simulink model "mrefrobotarm_modified_previous_y_previous_u_previous_ref_pert_2"  (R2018b)
settings: Solver=FixedStepAuto  StartTime=0.0  StopTime=60  RelTol=1e-3  AbsTol=1e-6
undefined symbols (not defined in the file or in its folder): cc, options
libraries: neural x858, simulink x1
(part 16 of 32)

== system mrefrobotarm_modified_previous_y_previous_u_previous_ref_pert_2/m=0 sd=0.1/Layer 3/Delays 1 ==
  "p{3}" : Inport  PortDimensions=30
      mask Display: e = 0.06;c1 = [120 230 180]/255;c2 = ([120 230 180]+0)/(256+128);c3 = ([120 230 180]+128)/(256+128);patch([0 1 1 0],[0 0 1 1],c1);patch([0 1 1 1-e 1-e 0+e],[0 0 1 1-e 0+e 0+e],c2);patch([0 0 1 1-e 0+e 0+e],[0 1 1 1-e 1-e 0+e],c3);plot([0 1 1 0 0],[0 0 1 1 0]);
  mux : Mux  Inputs=1
      mask Display: e = 0.06;c1 = [120 150 230]/255;c2 = ([120 150 230]+0)/383;c3 = ([120 150 230]+128)/383;patch([0 1 1 0],[0 0 1 1],c1);patch([0 1 1 1-e 1-e 0+e],[0 0 1 1-e 0+e 0+e],c2);patch([0 0 1 1-e 0+e 0+e],[0 1 1 1-e 1-e 0+e],c3);plot([0 1 1 0 0],[0 0 1 1 0]);disp('Mux')
  "pd{3,2}" : Outport
      mask Display: e = 0.06;c1 = [120 230 180]/255;c2 = ([120 230 180]+0)/(256+128);c3 = ([120 230 180]+128)/(256+128);patch([0 1 1 0],[0 0 1 1],c1);patch([0 1 1 1-e 1-e 0+e],[0 0 1 1-e 0+e 0+e],c2);patch([0 0 1 1-e 0+e 0+e],[0 1 1 1-e 1-e 0+e],c3);plot([0 1 1 0 0],[0 0 1 1 0]);
  wires:
  "p{3}"/1 -> mux/1
  mux/1 -> "pd{3,2}"/1

== system mrefrobotarm_modified_previous_y_previous_u_previous_ref_pert_2/m=0 sd=0.1/Layer 3/LW{3,2} ==
  "ad{3,2}" : Inport  PortDimensions=30
      mask Display: e = 0.06;c1 = [120 230 180]/255;c2 = ([120 230 180]+0)/(256+128);c3 = ([120 230 180]+128)/(256+128);patch([0 1 1 0],[0 0 1 1],c1);patch([0 1 1 1-e 1-e 0+e],[0 0 1 1-e 0+e 0+e],c2);patch([0 0 1 1-e 0+e 0+e],[0 1 1 1-e 1-e 0+e],c3);plot([0 1 1 0 0],[0 0 1 1 0]);
  "IW{3,2}(1,:)'" : Constant  Value=[0.55901254797417976316609156128834001719951629638671875;0.1893376853911200308200335484798415564000606536865234375;-0.0561053598569281330998848034141701646149158477783203125;0.006936116057090567499354705205405480228364467620849609375;0.10585635712547609987854713153865304775536060333251953125;-0.056411161009771886021280096201735432259738445281982421875;-0.362521364744238516752972145695821382105350494384765625;0.061274149008166800545183150461525656282901763916015625;-0.10299753787049596709390897331104497425258159637451171875;-1.0111912490182943802352610873640514910221099853515625;0.0080365135532425302500314501230604946613311767578125;0.038057999796948550896846796831596293486654758453369140625;0.0182019329420017549059362949037677026353776454925537109375;0.000718748845277970729687744277924821290071122348308563232421875;-0.0892154937366842204493622148220310918986797332763671875;0.04086688119049319833919753364170901477336883544921875;0.07794534518223993069252486520781530998647212982177734375;0.00118864659777381700793419394557304258341901004314422607421875;0.2021661306486308429253284657534095458686351776123046875;0.03908324016475679674176291200637933798134326934814453125;-0.088708253793172653356435830573900602757930755615234375;0.0043019444601169846975619037721116910688579082489013671875;-0.417578792656369823799167306788149289786815643310546875;0.0038865187767530167718688094424805967719294130802154541015625;-0.00952243697565639639346368738870296510867774486541748046875;0.416065824298875563957977874451898969709873199462890625;-0.1244373729702374087313643258312367834150791168212890625;0.021685469644277984013758242554104072041809558868408203125;-0.33337725597607625882545789863797836005687713623046875;-0.07267474571307540320841411585206515155732631683349609375]
      mask Display: e = 0.06;c1 = [120 150 230]/255;c2 = ([120 150 230]+0)/383;c3 = ([120 150 230]+128)/383;patch([0 1 1 0],[0 0 1 1],c1);patch([0 1 1 1-e 1-e 0+e],[0 0 1 1-e 0+e 0+e],c2);patch([0 0 1 1-e 0+e 0+e],[0 1 1 1-e 1-e 0+e],c3);plot([0 1 1 0 0],[0 0 1 1 0]);disp('weights');
  Mux : Mux  Inputs=1
      mask Display: e = 0.06;c1 = [120 150 230]/255;c2 = ([120 150 230]+0)/383;c3 = ([120 150 230]+128)/383;patch([0 1 1 0],[0 0 1 1],c1);patch([0 1 1 1-e 1-e 0+e],[0 0 1 1-e 0+e 0+e],c2);patch([0 0 1 1-e 0+e 0+e],[0 1 1 1-e 1-e 0+e],c3);plot([0 1 1 0 0],[0 0 1 1 0]);disp('Mux');
  dotprod1 : neural/Weight Functions/dotprod
  "lz{3,2}" : Outport
      mask Display: e = 0.06;c1 = [120 230 180]/255;c2 = ([120 230 180]+0)/(256+128);c3 = ([120 230 180]+128)/(256+128);patch([0 1 1 0],[0 0 1 1],c1);patch([0 1 1 1-e 1-e 0+e],[0 0 1 1-e 0+e 0+e],c2);patch([0 0 1 1-e 0+e 0+e],[0 1 1 1-e 1-e 0+e],c3);plot([0 1 1 0 0],[0 0 1 1 0]);
  wires:
  "IW{3,2}(1,:)'"/1 -> dotprod1/1
  "ad{3,2}"/1 -> dotprod1/2
  dotprod1/1 -> Mux/1
  Mux/1 -> "lz{3,2}"/1

== system mrefrobotarm_modified_previous_y_previous_u_previous_ref_pert_2/m=0 sd=0.2/Layer 1/Delays 1 ==
  "p{1}" : Inport  PortDimensions=10
      mask Display: e = 0.06;c1 = [120 230 180]/255;c2 = ([120 230 180]+0)/(256+128);c3 = ([120 230 180]+128)/(256+128);patch([0 1 1 0],[0 0 1 1],c1);patch([0 1 1 1-e 1-e 0+e],[0 0 1 1-e 0+e 0+e],c2);patch([0 0 1 1-e 0+e 0+e],[0 1 1 1-e 1-e 0+e],c3);plot([0 1 1 0 0],[0 0 1 1 0]);
  mux : Mux  Inputs=1
      mask Display: e = 0.06;c1 = [120 150 230]/255;c2 = ([120 150 230]+0)/383;c3 = ([120 150 230]+128)/383;patch([0 1 1 0],[0 0 1 1],c1);patch([0 1 1 1-e 1-e 0+e],[0 0 1 1-e 0+e 0+e],c2);patch([0 0 1 1-e 0+e 0+e],[0 1 1 1-e 1-e 0+e],c3);plot([0 1 1 0 0],[0 0 1 1 0]);disp('Mux')
  "pd{1,1}" : Outport
      mask Display: e = 0.06;c1 = [120 230 180]/255;c2 = ([120 230 180]+0)/(256+128);c3 = ([120 230 180]+128)/(256+128);patch([0 1 1 0],[0 0 1 1],c1);patch([0 1 1 1-e 1-e 0+e],[0 0 1 1-e 0+e 0+e],c2);patch([0 0 1 1-e 0+e 0+e],[0 1 1 1-e 1-e 0+e],c3);plot([0 1 1 0 0],[0 0 1 1 0]);
  wires:
  "p{1}"/1 -> mux/1
  mux/1 -> "pd{1,1}"/1

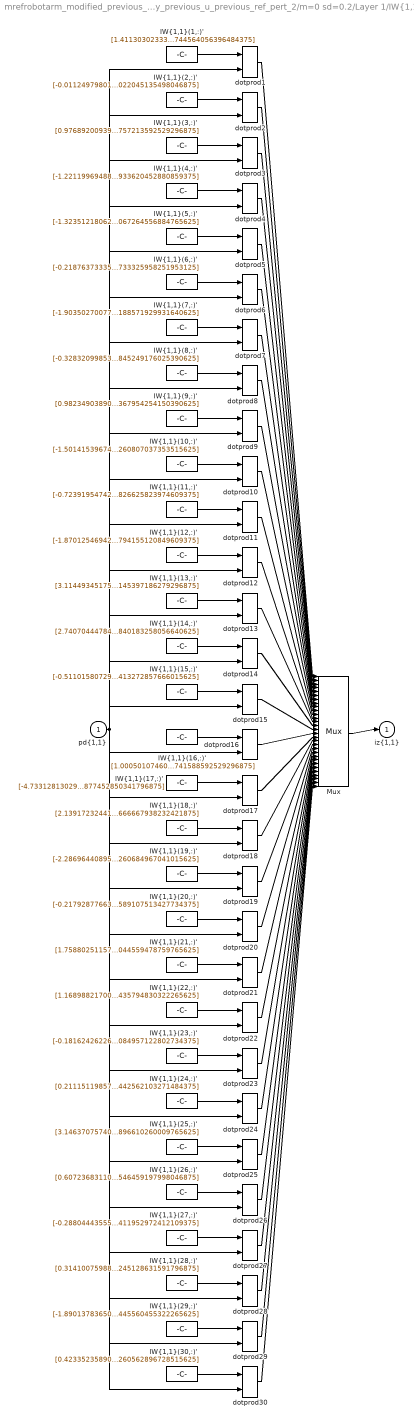
== system mrefrobotarm_modified_previous_y_previous_u_previous_ref_pert_2/m=0 sd=0.2/Layer 1/IW{1,1} ==
  "pd{1,1}" : Inport  PortDimensions=10
      mask Display: e = 0.06;c1 = [120 230 180]/255;c2 = ([120 230 180]+0)/(256+128);c3 = ([120 230 180]+128)/(256+128);patch([0 1 1 0],[0 0 1 1],c1);patch([0 1 1 1-e 1-e 0+e],[0 0 1 1-e 0+e 0+e],c2);patch([0 0 1 1-e 0+e 0+e],[0 1 1 1-e 1-e 0+e],c3);plot([0 1 1 0 0],[0 0 1 1 0]);
  "IW{1,1}(1,:)'" : Constant  Value=[1.4113030233343781816301998333074152469635009765625;-0.348438589909515428200137421299587003886699676513671875;-1.525310697435914963904224350699223577976226806640625;0.2209845967001718702871215782579383812844753265380859375;-0.90644875404291724851901790316333062946796417236328125;3.15955488668658812656531154061667621135711669921875;-1.645213986417652929361565838917158544063568115234375;0.31425769225662125716524997187661938369274139404296875;5.8448616430047390934987561195157468318939208984375;2.639470335514532361997908083139918744564056396484375]
      mask Display: e = 0.06;c1 = [120 150 230]/255;c2 = ([120 150 230]+0)/383;c3 = ([120 150 230]+128)/383;patch([0 1 1 0],[0 0 1 1],c1);patch([0 1 1 1-e 1-e 0+e],[0 0 1 1-e 0+e 0+e],c2);patch([0 0 1 1-e 0+e 0+e],[0 1 1 1-e 1-e 0+e],c3);plot([0 1 1 0 0],[0 0 1 1 0]);disp('Weights');
  "IW{1,1}(10,:)'" : Constant  Value=[-1.5014153967441250525638452018029056489467620849609375;0.9736603972080974944702802531537599861621856689453125;-1.37313114935890911993965346482582390308380126953125;0.453944962788460470992646378363133408129215240478515625;-0.517586043869458389821147648035548627376556396484375;0.86773315026872366306776029887259937822818756103515625;-0.11243588136571429358934182118900935165584087371826171875;0.539938227324440855880993694881908595561981201171875;0.6911668193214997035767055422184057533740997314453125;-0.034160834851410117052328274667161167599260807037353515625]
      mask Display: e = 0.06;c1 = [120 150 230]/255;c2 = ([120 150 230]+0)/383;c3 = ([120 150 230]+128)/383;patch([0 1 1 0],[0 0 1 1],c1);patch([0 1 1 1-e 1-e 0+e],[0 0 1 1-e 0+e 0+e],c2);patch([0 0 1 1-e 0+e 0+e],[0 1 1 1-e 1-e 0+e],c3);plot([0 1 1 0 0],[0 0 1 1 0]);disp('Weights');
  "IW{1,1}(11,:)'" : Constant  Value=[-0.72391954742164899005985034818877466022968292236328125;0.60057208214730983808493647302384488284587860107421875;-1.4507267854128438333560779938125051558017730712890625;0.456866710462218217347896143110119737684726715087890625;0.1570974108836583338355552541543147526681423187255859375;0.733544275114982990970702303457073867321014404296875;-0.598466107260065438566698503564111888408660888671875;-0.480699831251547526900225193458027206361293792724609375;2.35513038112840877857934174244292080402374267578125;1.419047822295259830838176640099845826625823974609375]
      mask Display: e = 0.06;c1 = [120 150 230]/255;c2 = ([120 150 230]+0)/383;c3 = ([120 150 230]+128)/383;patch([0 1 1 0],[0 0 1 1],c1);patch([0 1 1 1-e 1-e 0+e],[0 0 1 1-e 0+e 0+e],c2);patch([0 0 1 1-e 0+e 0+e],[0 1 1 1-e 1-e 0+e],c3);plot([0 1 1 0 0],[0 0 1 1 0]);disp('Weights');
  "IW{1,1}(12,:)'" : Constant  Value=[-1.87012546942036284036703364108689129352569580078125;1.3084444749908488159206854106741957366466522216796875;-1.1877577962136418587846264927065931260585784912109375;1.2551744503796522511862576720886863768100738525390625;0.11790915105610698387916812635012320242822170257568359375;-0.4054577111017920731939057077397592365741729736328125;0.86175101157558942066572171825100667774677276611328125;0.84046199333763393912732908574980683624744415283203125;-1.552570172382738977745475494884885847568511962890625;-0.8322997096343731637801965916878543794155120849609375]
      mask Display: e = 0.06;c1 = [120 150 230]/255;c2 = ([120 150 230]+0)/383;c3 = ([120 150 230]+128)/383;patch([0 1 1 0],[0 0 1 1],c1);patch([0 1 1 1-e 1-e 0+e],[0 0 1 1-e 0+e 0+e],c2);patch([0 0 1 1-e 0+e 0+e],[0 1 1 1-e 1-e 0+e],c3);plot([0 1 1 0 0],[0 0 1 1 0]);disp('Weights');
  "IW{1,1}(13,:)'" : Constant  Value=[3.11449345175705349930694865179248154163360595703125;-3.732348373191891166555933523341082036495208740234375;-0.6723234936499988823044304808718152344226837158203125;1.0218838198423327856545483882655389606952667236328125;0.1369109814135320013495089597199694253504276275634765625;-0.76304172975338036000181318740942515432834625244140625;0.7623366887407232450613037144648842513561248779296875;1.02980844388660042199035160592757165431976318359375;-3.248414372584246923025830255937762558460235595703125;-2.232600966299432609929453974473290145397186279296875]
      mask Display: e = 0.06;c1 = [120 150 230]/255;c2 = ([120 150 230]+0)/383;c3 = ([120 150 230]+128)/383;patch([0 1 1 0],[0 0 1 1],c1);patch([0 1 1 1-e 1-e 0+e],[0 0 1 1-e 0+e 0+e],c2);patch([0 0 1 1-e 0+e 0+e],[0 1 1 1-e 1-e 0+e],c3);plot([0 1 1 0 0],[0 0 1 1 0]);disp('Weights');
  "IW{1,1}(14,:)'" : Constant  Value=[2.74070444784985323138926105457358062267303466796875;-2.820073129625178420809561430360190570354461669921875;-1.1487312568141889723705162396072410047054290771484375;0.088073813383340804339383112164796330034732818603515625;0.49531928111860723529247252372442744672298431396484375;3.474324634455964844192976670456118881702423095703125;-2.657024722837350250159715869813226163387298583984375;-0.0478319365917047878422607709580915980041027069091796875;4.809776553517846053864559507928788661956787109375;5.53419618962490122981989770778454840183258056640625]
      mask Display: e = 0.06;c1 = [120 150 230]/255;c2 = ([120 150 230]+0)/383;c3 = ([120 150 230]+128)/383;patch([0 1 1 0],[0 0 1 1],c1);patch([0 1 1 1-e 1-e 0+e],[0 0 1 1-e 0+e 0+e],c2);patch([0 0 1 1-e 0+e 0+e],[0 1 1 1-e 1-e 0+e],c3);plot([0 1 1 0 0],[0 0 1 1 0]);disp('Weights');
  "IW{1,1}(15,:)'" : Constant  Value=[-0.511015807291060664141468805610202252864837646484375;-0.347029031123842646167076964047737419605255126953125;-0.1718418816922243907985290434226044453680515289306640625;0.55723542002860548816300934049650095403194427490234375;1.001218620463129038711258544935844838619232177734375;0.5480449416585952970848438781104050576686859130859375;-1.2905089839227572579005709485500119626522064208984375;-0.311064951952224777453892556877690367400646209716796875;1.605461938449392444994145989767275750637054443359375;0.57757524693824591199842188871116377413272857666015625]
      mask Display: e = 0.06;c1 = [120 150 230]/255;c2 = ([120 150 230]+0)/383;c3 = ([120 150 230]+128)/383;patch([0 1 1 0],[0 0 1 1],c1);patch([0 1 1 1-e 1-e 0+e],[0 0 1 1-e 0+e 0+e],c2);patch([0 0 1 1-e 0+e 0+e],[0 1 1 1-e 1-e 0+e],c3);plot([0 1 1 0 0],[0 0 1 1 0]);disp('Weights');
  "IW{1,1}(16,:)'" : Constant  Value=[1.000501074609136065163284001755528151988983154296875;-0.71026830395794637862394438343471847474575042724609375;0.56643772389824775803646161875803954899311065673828125;-1.718593345145298822984614162123762071132659912109375;-0.04658830456743641434957936553473700769245624542236328125;1.896992873999785000904694243217818439006805419921875;-1.314207523734456817265936479088850319385528564453125;-0.58100817248522618196915345833986066281795501708984375;6.11342037772077606661014215205796062946319580078125;4.26490922194190869021213075029663741588592529296875]
      mask Display: e = 0.06;c1 = [120 150 230]/255;c2 = ([120 150 230]+0)/383;c3 = ([120 150 230]+128)/383;patch([0 1 1 0],[0 0 1 1],c1);patch([0 1 1 1-e 1-e 0+e],[0 0 1 1-e 0+e 0+e],c2);patch([0 0 1 1-e 0+e 0+e],[0 1 1 1-e 1-e 0+e],c3);plot([0 1 1 0 0],[0 0 1 1 0]);disp('Weights');
  "IW{1,1}(17,:)'" : Constant  Value=[-4.73312813029816314980280367308296263217926025390625;6.01312541072434303401905708597041666507720947265625;0.1446975706664820615632294220631592907011508941650390625;-1.3734916538271806363269433859386481344699859619140625;-0.374570868930040601352260409839800558984279632568359375;-6.0102833405435394098503820714540779590606689453125;5.72011522082058210258992403396405279636383056640625;0.129537853146572012885684443972422741353511810302734375;-17.05733403236849454742696252651512622833251953125;-12.2512694254419596262550840037874877452850341796875]
      mask Display: e = 0.06;c1 = [120 150 230]/255;c2 = ([120 150 230]+0)/383;c3 = ([120 150 230]+128)/383;patch([0 1 1 0],[0 0 1 1],c1);patch([0 1 1 1-e 1-e 0+e],[0 0 1 1-e 0+e 0+e],c2);patch([0 0 1 1-e 0+e 0+e],[0 1 1 1-e 1-e 0+e],c3);plot([0 1 1 0 0],[0 0 1 1 0]);disp('Weights');
  "IW{1,1}(18,:)'" : Constant  Value=[2.139172324417781823058248846791684627532958984375;-1.516704379288808635095620047650299966335296630859375;-0.97354754756783012936693921801634132862091064453125;2.15205674059551288479497088701464235782623291015625;-1.16111579032775669162447229609824717044830322265625;-1.30932797370402465020333693246357142925262451171875;0.4970822382713446785373889724723994731903076171875;0.003946372609830076268189191779356406186707317829132080078125;-1.6373923459250760981120720316539518535137176513671875;-0.876724016447773646376617762143723666667938232421875]
      mask Display: e = 0.06;c1 = [120 150 230]/255;c2 = ([120 150 230]+0)/383;c3 = ([120 150 230]+128)/383;patch([0 1 1 0],[0 0 1 1],c1);patch([0 1 1 1-e 1-e 0+e],[0 0 1 1-e 0+e 0+e],c2);patch([0 0 1 1-e 0+e 0+e],[0 1 1 1-e 1-e 0+e],c3);plot([0 1 1 0 0],[0 0 1 1 0]);disp('Weights');
  "IW{1,1}(19,:)'" : Constant  Value=[-2.2869644089557112920374493114650249481201171875;2.06966810652304555873115532449446618556976318359375;1.90142951742451060681560193188488483428955078125;-0.574308612498034332105589783168397843837738037109375;-0.247708051032199449981163752454449422657489776611328125;0.5564187144200676282679296491551212966442108154296875;-1.56539549833531221878502037725411355495452880859375;0.375078818331078533976352673562359996140003204345703125;2.397843513239210633258835514425300061702728271484375;1.3119695913197606529365657479502260684967041015625]
      mask Display: e = 0.06;c1 = [120 150 230]/255;c2 = ([120 150 230]+0)/383;c3 = ([120 150 230]+128)/383;patch([0 1 1 0],[0 0 1 1],c1);patch([0 1 1 1-e 1-e 0+e],[0 0 1 1-e 0+e 0+e],c2);patch([0 0 1 1-e 0+e 0+e],[0 1 1 1-e 1-e 0+e],c3);plot([0 1 1 0 0],[0 0 1 1 0]);disp('Weights');
  "IW{1,1}(2,:)'" : Constant  Value=[-0.0112497980128958285916951354010961949825286865234375;0.06194588216941789016178887550267972983419895172119140625;0.5652958623659614101342185676912777125835418701171875;-1.180785608869924896424663529614917933940887451171875;0.088823412488288344679432384509709663689136505126953125;2.13880595730649947228130258736200630664825439453125;-2.27945305012616472595254890620708465576171875;0.281685433695026576916831118069239892065525054931640625;4.35874409348693614418834840762428939342498779296875;3.18642541802911960502342481049709022045135498046875]
      mask Display: e = 0.06;c1 = [120 150 230]/255;c2 = ([120 150 230]+0)/383;c3 = ([120 150 230]+128)/383;patch([0 1 1 0],[0 0 1 1],c1);patch([0 1 1 1-e 1-e 0+e],[0 0 1 1-e 0+e 0+e],c2);patch([0 0 1 1-e 0+e 0+e],[0 1 1 1-e 1-e 0+e],c3);plot([0 1 1 0 0],[0 0 1 1 0]);disp('Weights');
  "IW{1,1}(20,:)'" : Constant  Value=[-0.217928776638212584604303856394835747778415679931640625;0.40520405266274883704369358383701182901859283447265625;-0.04396564242946267297984519473175168968737125396728515625;-0.043313894632832923570209260333285783417522907257080078125;-0.045148919419630346994143366146090556867420673370361328125;-0.2359067249724053905168830169714055955410003662109375;0.09766924760321415988073567859828472137451171875;0.0686057321137425735191328612927463836967945098876953125;-0.35078030086031863898909932686365209519863128662109375;-0.3633796929059707192521955221309326589107513427734375]
      mask Display: e = 0.06;c1 = [120 150 230]/255;c2 = ([120 150 230]+0)/383;c3 = ([120 150 230]+128)/383;patch([0 1 1 0],[0 0 1 1],c1);patch([0 1 1 1-e 1-e 0+e],[0 0 1 1-e 0+e 0+e],c2);patch([0 0 1 1-e 0+e 0+e],[0 1 1 1-e 1-e 0+e],c3);plot([0 1 1 0 0],[0 0 1 1 0]);disp('Weights');
  "IW{1,1}(21,:)'" : Constant  Value=[1.7588025115735634873459503069170750677585601806640625;-2.282420941548847448387959957472048699855804443359375;-1.0294915097698116301927484528278000652790069580078125;1.8482290099310336728422043961472809314727783203125;-0.2097696977909766780090450311035965569317340850830078125;-1.9311459400257862117911145105608738958835601806640625;3.31019261230273986740257896599359810352325439453125;-0.417497660482693933037268152475007809698581695556640625;-7.56322499549997484535879266331903636455535888671875;-4.4413848237048316747177523211576044559478759765625]
      mask Display: e = 0.06;c1 = [120 150 230]/255;c2 = ([120 150 230]+0)/383;c3 = ([120 150 230]+128)/383;patch([0 1 1 0],[0 0 1 1],c1);patch([0 1 1 1-e 1-e 0+e],[0 0 1 1-e 0+e 0+e],c2);patch([0 0 1 1-e 0+e 0+e],[0 1 1 1-e 1-e 0+e],c3);plot([0 1 1 0 0],[0 0 1 1 0]);disp('Weights');
  "IW{1,1}(22,:)'" : Constant  Value=[1.168988217006086127724984180531464517116546630859375;-1.732957486285161774475227502989582717418670654296875;1.05320711434076752510691221687011420726776123046875;-0.58838238416820487497460590020637027919292449951171875;1.3083920626301372980293535874807275831699371337890625;1.3241783743371711157266190639347769320011138916015625;-0.6789672752525373056187163456343114376068115234375;-0.05675259587550791906540581521767308004200458526611328125;1.7931659248481632840110933102550916373729705810546875;1.2789209238231313836564595476374961435794830322265625]
      mask Display: e = 0.06;c1 = [120 150 230]/255;c2 = ([120 150 230]+0)/383;c3 = ([120 150 230]+128)/383;patch([0 1 1 0],[0 0 1 1],c1);patch([0 1 1 1-e 1-e 0+e],[0 0 1 1-e 0+e 0+e],c2);patch([0 0 1 1-e 0+e 0+e],[0 1 1 1-e 1-e 0+e],c3);plot([0 1 1 0 0],[0 0 1 1 0]);disp('Weights');
  "IW{1,1}(23,:)'" : Constant  Value=[-0.1816242622647597226848148466160637326538562774658203125;0.404100028294180513288580414155148901045322418212890625;0.81985447175648629158928315519005991518497467041015625;0.446234395527585092633415797536144964396953582763671875;-0.06698452232360314895220909647832741029560565948486328125;-0.67328712640305587999733916149125434458255767822265625;0.0986983678558296662064464044306077994406223297119140625;0.024026327828121300800301440858675050549209117889404296875;0.055343344102837692399798896758511546067893505096435546875;1.0238225121892321478611620477749966084957122802734375]
      mask Display: e = 0.06;c1 = [120 150 230]/255;c2 = ([120 150 230]+0)/383;c3 = ([120 150 230]+128)/383;patch([0 1 1 0],[0 0 1 1],c1);patch([0 1 1 1-e 1-e 0+e],[0 0 1 1-e 0+e 0+e],c2);patch([0 0 1 1-e 0+e 0+e],[0 1 1 1-e 1-e 0+e],c3);plot([0 1 1 0 0],[0 0 1 1 0]);disp('Weights');
  "IW{1,1}(24,:)'" : Constant  Value=[0.2111511985769846944105410102565656416118144989013671875;-0.65549437434372237465396437983145006000995635986328125;-2.394869521885237606539931221050210297107696533203125;1.7365146143944210077592060770257376134395599365234375;-0.7276256124627735744070378132164478302001953125;1.0356434790147996949372100061737000942230224609375;-0.57912371388859906762291984705370850861072540283203125;-0.413357730849843785225772307967417873442173004150390625;2.76287761606681225856618766556493937969207763671875;2.773418915272047424736001630662940442562103271484375]
      mask Display: e = 0.06;c1 = [120 150 230]/255;c2 = ([120 150 230]+0)/383;c3 = ([120 150 230]+128)/383;patch([0 1 1 0],[0 0 1 1],c1);patch([0 1 1 1-e 1-e 0+e],[0 0 1 1-e 0+e 0+e],c2);patch([0 0 1 1-e 0+e 0+e],[0 1 1 1-e 1-e 0+e],c3);plot([0 1 1 0 0],[0 0 1 1 0]);disp('Weights');
  "IW{1,1}(25,:)'" : Constant  Value=[3.1463707574085528761997920810244977474212646484375;-4.5461189975282092490260765771381556987762451171875;0.51061308134607441555630202856264077126979827880859375;0.71238199390895318163785532306064851582050323486328125;1.2749205388401552152544127238797955214977264404296875;-3.515132059874350733963410675642080605030059814453125;2.022847367905899584883400166290812194347381591796875;-0.65197883673105450075269118315191008150577545166015625;-5.002664971606190391639756853692233562469482421875;-4.67685034405227018083905932144261896610260009765625]
      mask Display: e = 0.06;c1 = [120 150 230]/255;c2 = ([120 150 230]+0)/383;c3 = ([120 150 230]+128)/383;patch([0 1 1 0],[0 0 1 1],c1);patch([0 1 1 1-e 1-e 0+e],[0 0 1 1-e 0+e 0+e],c2);patch([0 0 1 1-e 0+e 0+e],[0 1 1 1-e 1-e 0+e],c3);plot([0 1 1 0 0],[0 0 1 1 0]);disp('Weights');
  "IW{1,1}(26,:)'" : Constant  Value=[0.60723683110464021783769794637919403612613677978515625;-1.03930083857456256879459033370949327945709228515625;0.128013863473342370813412571806111373007297515869140625;-0.021256590523661321456838635413078009150922298431396484375;0.5014674643389636088386396295391023159027099609375;-0.025097806043500807404722507953920285217463970184326171875;0.0110005865361357986487167437417156179435551166534423828125;-0.1261370054402988216679659672081470489501953125;0.27395045669768591789505762790213339030742645263671875;-0.04029258447016641209170728643584880046546459197998046875]
      mask Display: e = 0.06;c1 = [120 150 230]/255;c2 = ([120 150 230]+0)/383;c3 = ([120 150 230]+128)/383;patch([0 1 1 0],[0 0 1 1],c1);patch([0 1 1 1-e 1-e 0+e],[0 0 1 1-e 0+e 0+e],c2);patch([0 0 1 1-e 0+e 0+e],[0 1 1 1-e 1-e 0+e],c3);plot([0 1 1 0 0],[0 0 1 1 0]);disp('Weights');
  "IW{1,1}(27,:)'" : Constant  Value=[-0.288044435559366041044171424800879321992397308349609375;-0.31773988771733685521070356116979382932186126708984375;-0.4960175697311510756293273516348563134670257568359375;1.3154389797310239718086677385144867002964019775390625;-1.8929129505798261146054528580862097442150115966796875;0.72651386866147615872790765934041701257228851318359375;-2.457680099152586450372837134636938571929931640625;-0.1317981758047972740133246816185419447720050811767578125;3.252378072760266025653663746197707951068878173828125;1.9785481281466521519263324080384336411952972412109375]
      mask Display: e = 0.06;c1 = [120 150 230]/255;c2 = ([120 150 230]+0)/383;c3 = ([120 150 230]+128)/383;patch([0 1 1 0],[0 0 1 1],c1);patch([0 1 1 1-e 1-e 0+e],[0 0 1 1-e 0+e 0+e],c2);patch([0 0 1 1-e 0+e 0+e],[0 1 1 1-e 1-e 0+e],c3);plot([0 1 1 0 0],[0 0 1 1 0]);disp('Weights');
  "IW{1,1}(28,:)'" : Constant  Value=[0.31410075988516350520285413949750363826751708984375;1.581538030292237717588932355283759534358978271484375;0.91703733056539549206576111828326247632503509521484375;-2.5035969635325319160301660303957760334014892578125;-1.796199207869567882056571761495433747768402099609375;1.36595065376107438481767530902288854122161865234375;-0.09586923444364987834109825826089945621788501739501953125;1.0122978981203007986522379724192433059215545654296875;1.185094962913229910128620758769102394580841064453125;1.122283111931022148155534523539245128631591796875]
      mask Display: e = 0.06;c1 = [120 150 230]/255;c2 = ([120 150 230]+0)/383;c3 = ([120 150 230]+128)/383;patch([0 1 1 0],[0 0 1 1],c1);patch([0 1 1 1-e 1-e 0+e],[0 0 1 1-e 0+e 0+e],c2);patch([0 0 1 1-e 0+e 0+e],[0 1 1 1-e 1-e 0+e],c3);plot([0 1 1 0 0],[0 0 1 1 0]);disp('Weights');
  "IW{1,1}(29,:)'" : Constant  Value=[-1.890137836503250401420928028528578579425811767578125;0.30590264537788891541225666514947079122066497802734375;0.457178412451843596553402448989800177514553070068359375;0.632323839291558886799293759395368397235870361328125;0.56627061986790738767894026750582270324230194091796875;1.7675189571870404403597376585821621119976043701171875;-1.5379864412138732898682746963459067046642303466796875;-0.2118306249555119702421279725967906415462493896484375;6.42448474301508998252074889023788273334503173828125;4.6108162037688860124262646422721445560455322265625]
      mask Display: e = 0.06;c1 = [120 150 230]/255;c2 = ([120 150 230]+0)/383;c3 = ([120 150 230]+128)/383;patch([0 1 1 0],[0 0 1 1],c1);patch([0 1 1 1-e 1-e 0+e],[0 0 1 1-e 0+e 0+e],c2);patch([0 0 1 1-e 0+e 0+e],[0 1 1 1-e 1-e 0+e],c3);plot([0 1 1 0 0],[0 0 1 1 0]);disp('Weights');
  "IW{1,1}(3,:)'" : Constant  Value=[0.97689200939192677441980094954487867653369903564453125;-2.1538424162847089604611028335057199001312255859375;0.26140280744923583000627331784926354885101318359375;-0.1605118486471729666309471440399647690355777740478515625;0.1045633614604802030800811962762963958084583282470703125;1.712121135219027312501793858245946466922760009765625;-1.380113117190847393800368081429041922092437744140625;-0.62423621411588559038108314780401997268199920654296875;5.89567838099284102781894034706056118011474609375;3.406453311621791879559850713121704757213592529296875]
      mask Display: e = 0.06;c1 = [120 150 230]/255;c2 = ([120 150 230]+0)/383;c3 = ([120 150 230]+128)/383;patch([0 1 1 0],[0 0 1 1],c1);patch([0 1 1 1-e 1-e 0+e],[0 0 1 1-e 0+e 0+e],c2);patch([0 0 1 1-e 0+e 0+e],[0 1 1 1-e 1-e 0+e],c3);plot([0 1 1 0 0],[0 0 1 1 0]);disp('Weights');
  "IW{1,1}(30,:)'" : Constant  Value=[0.42335235890965139393671279322006739675998687744140625;-0.17019253965468517098003076171153225004673004150390625;0.29055996237503778356625616652308963239192962646484375;-0.57204890245736972342882609154912643134593963623046875;-1.0126167177395026808284228536649607121944427490234375;1.9495388602539491795795356665621511638164520263671875;-0.844271742393967183915037821861915290355682373046875;0.0719968818419344513959146070192218758165836334228515625;1.632735464634091027136264528962783515453338623046875;2.390729933131736206775030950666405260562896728515625]
      mask Display: e = 0.06;c1 = [120 150 230]/255;c2 = ([120 150 230]+0)/383;c3 = ([120 150 230]+128)/383;patch([0 1 1 0],[0 0 1 1],c1);patch([0 1 1 1-e 1-e 0+e],[0 0 1 1-e 0+e 0+e],c2);patch([0 0 1 1-e 0+e 0+e],[0 1 1 1-e 1-e 0+e],c3);plot([0 1 1 0 0],[0 0 1 1 0]);disp('Weights');
  "IW{1,1}(4,:)'" : Constant  Value=[-1.22119969488670943036368043976835906505584716796875;1.16885618554226056176048587076365947723388671875;-0.72338987562096779271314517245627939701080322265625;1.122032623546176832718401783495210111141204833984375;-2.117249178777793616745839244686067104339599609375;-1.3230034459321531326025933594792149960994720458984375;-0.36698636920591243271161374650546349585056304931640625;0.08206546644491950759370268997372477315366268157958984375;-1.874481097167512988477255930774845182895660400390625;-1.843374971515357341189655926427803933620452880859375]
      mask Display: e = 0.06;c1 = [120 150 230]/255;c2 = ([120 150 230]+0)/383;c3 = ([120 150 230]+128)/383;patch([0 1 1 0],[0 0 1 1],c1);patch([0 1 1 1-e 1-e 0+e],[0 0 1 1-e 0+e 0+e],c2);patch([0 0 1 1-e 0+e 0+e],[0 1 1 1-e 1-e 0+e],c3);plot([0 1 1 0 0],[0 0 1 1 0]);disp('Weights');
  "IW{1,1}(5,:)'" : Constant  Value=[-1.3235121806255103482641288792365230619907379150390625;3.29187147790517098400187023798935115337371826171875;0.31934110466331977473686265511787496507167816162109375;-1.6336042355737807607596323578036390244960784912109375;-1.3137603245591564782301929881214164197444915771484375;-1.845325062076014877021634674747474491596221923828125;2.4908796928078391630378973786719143390655517578125;0.04047302533535117319285490111724357120692729949951171875;-4.87710765674354274068491577054373919963836669921875;-3.31950636347878091925167609588243067264556884765625]
      mask Display: e = 0.06;c1 = [120 150 230]/255;c2 = ([120 150 230]+0)/383;c3 = ([120 150 230]+128)/383;patch([0 1 1 0],[0 0 1 1],c1);patch([0 1 1 1-e 1-e 0+e],[0 0 1 1-e 0+e 0+e],c2);patch([0 0 1 1-e 0+e 0+e],[0 1 1 1-e 1-e 0+e],c3);plot([0 1 1 0 0],[0 0 1 1 0]);disp('Weights');
  "IW{1,1}(6,:)'" : Constant  Value=[-0.21876373335746623904896068779635243117809295654296875;1.6989450640047485396877391394809819757938385009765625;-0.84611335077068761112428774140425957739353179931640625;0.1653387842750385916534838770530768670141696929931640625;-0.05095766038839720513120568057274795137345790863037109375;0.98579287932315329268107007010257802903652191162109375;-2.224886605820195040195130786742083728313446044921875;0.018838494904783238681478252374290605075657367706298828125;3.02041143717368498755604377947747707366943359375;1.2216980084773727543989707555738277733325958251953125]
      mask Display: e = 0.06;c1 = [120 150 230]/255;c2 = ([120 150 230]+0)/383;c3 = ([120 150 230]+128)/383;patch([0 1 1 0],[0 0 1 1],c1);patch([0 1 1 1-e 1-e 0+e],[0 0 1 1-e 0+e 0+e],c2);patch([0 0 1 1-e 0+e 0+e],[0 1 1 1-e 1-e 0+e],c3);plot([0 1 1 0 0],[0 0 1 1 0]);disp('Weights');
  "IW{1,1}(7,:)'" : Constant  Value=[-1.9035027007753118066801789609598927199840545654296875;3.278865573910130226664705332950688898563385009765625;-0.71428146077050858053780757472850382328033447265625;0.27895396863435462098124162366730161011219024658203125;-0.89989554860000708913503331132233142852783203125;0.1265448626848791058296939127103541977703571319580078125;-0.08459651118240486822319468274145037867128849029541015625;0.08194144685369997294088761918828822672367095947265625;0.512374197097207773055060897604562342166900634765625;0.8050294878008517063250337741919793188571929931640625]
      mask Display: e = 0.06;c1 = [120 150 230]/255;c2 = ([120 150 230]+0)/383;c3 = ([120 150 230]+128)/383;patch([0 1 1 0],[0 0 1 1],c1);patch([0 1 1 1-e 1-e 0+e],[0 0 1 1-e 0+e 0+e],c2);patch([0 0 1 1-e 0+e 0+e],[0 1 1 1-e 1-e 0+e],c3);plot([0 1 1 0 0],[0 0 1 1 0]);disp('Weights');
  "IW{1,1}(8,:)'" : Constant  Value=[-0.328320998530186314301460015485645271837711334228515625;0.60579099460622476414073389605619013309478759765625;-0.0913512880482287015215803194223553873598575592041015625;-0.058750623543463838249767405841339495964348316192626953125;-0.1469601123322662183934284030328853987157344818115234375;-0.35734534390833239125839781991089694201946258544921875;0.2491678549746647319818038113226066343486309051513671875;0.11173335160234720841998523610527627170085906982421875;-1.242725509484667867354801273904740810394287109375;-0.91232302728842251671181884375982917845249176025390625]
      mask Display: e = 0.06;c1 = [120 150 230]/255;c2 = ([120 150 230]+0)/383;c3 = ([120 150 230]+128)/383;patch([0 1 1 0],[0 0 1 1],c1);patch([0 1 1 1-e 1-e 0+e],[0 0 1 1-e 0+e 0+e],c2);patch([0 0 1 1-e 0+e 0+e],[0 1 1 1-e 1-e 0+e],c3);plot([0 1 1 0 0],[0 0 1 1 0]);disp('Weights');
  "IW{1,1}(9,:)'" : Constant  Value=[0.982349038906586979891244482132606208324432373046875;-0.6144818415170310021977684300509281456470489501953125;2.05158480497812689691272680647671222686767578125;-0.452979095340528215007935841640573926270008087158203125;0.750670639433560271669421126716770231723785400390625;-2.996784172537360291244112886488437652587890625;1.832004854111751068757030225242488086223602294921875;-0.691060865019840431244801948196254670619964599609375;-5.31554056911627537118647524039261043071746826171875;-2.972329136331547605465175365679897367954254150390625]
      mask Display: e = 0.06;c1 = [120 150 230]/255;c2 = ([120 150 230]+0)/383;c3 = ([120 150 230]+128)/383;patch([0 1 1 0],[0 0 1 1],c1);patch([0 1 1 1-e 1-e 0+e],[0 0 1 1-e 0+e 0+e],c2);patch([0 0 1 1-e 0+e 0+e],[0 1 1 1-e 1-e 0+e],c3);plot([0 1 1 0 0],[0 0 1 1 0]);disp('Weights');
  Mux : Mux  Inputs=30
      mask Display: e = 0.06;c1 = [120 150 230]/255;c2 = ([120 150 230]+0)/383;c3 = ([120 150 230]+128)/383;patch([0 1 1 0],[0 0 1 1],c1);patch([0 1 1 1-e 1-e 0+e],[0 0 1 1-e 0+e 0+e],c2);patch([0 0 1 1-e 0+e 0+e],[0 1 1 1-e 1-e 0+e],c3);plot([0 1 1 0 0],[0 0 1 1 0]);disp('Mux');
  dotprod{1..30} (30 alike) : neural/Weight Functions/dotprod
  "iz{1,1}" : Outport
      mask Display: e = 0.06;c1 = [120 230 180]/255;c2 = ([120 230 180]+0)/(256+128);c3 = ([120 230 180]+128)/(256+128);patch([0 1 1 0],[0 0 1 1],c1);patch([0 1 1 1-e 1-e 0+e],[0 0 1 1-e 0+e 0+e],c2);patch([0 0 1 1-e 0+e 0+e],[0 1 1 1-e 1-e 0+e],c3);plot([0 1 1 0 0],[0 0 1 1 0]);
  wires:
  "IW{1,1}(1,:)'"/1 -> dotprod1/1
  "pd{1,1}"/1 -> dotprod1/2, dotprod2/2, dotprod3/2, dotprod4/2, dotprod5/2, dotprod6/2, dotprod7/2, dotprod8/2, dotprod9/2, dotprod10/2, dotprod11/2, dotprod12/2, dotprod13/2, dotprod14/2, dotprod15/2, dotprod16/2, dotprod17/2, dotprod18/2, dotprod19/2, dotprod20/2, dotprod21/2, dotprod22/2, dotprod23/2, dotprod24/2, dotprod25/2, dotprod26/2, dotprod27/2, dotprod28/2, dotprod29/2, dotprod30/2
  dotprod1/1 -> Mux/1
  "IW{1,1}(2,:)'"/1 -> dotprod2/1
  dotprod2/1 -> Mux/2
  "IW{1,1}(3,:)'"/1 -> dotprod3/1
  dotprod3/1 -> Mux/3
  "IW{1,1}(4,:)'"/1 -> dotprod4/1
  dotprod4/1 -> Mux/4
  "IW{1,1}(5,:)'"/1 -> dotprod5/1
  dotprod5/1 -> Mux/5
  "IW{1,1}(6,:)'"/1 -> dotprod6/1
  dotprod6/1 -> Mux/6
  "IW{1,1}(7,:)'"/1 -> dotprod7/1
  dotprod7/1 -> Mux/7
  "IW{1,1}(8,:)'"/1 -> dotprod8/1
  dotprod8/1 -> Mux/8
  "IW{1,1}(9,:)'"/1 -> dotprod9/1
  dotprod9/1 -> Mux/9
  "IW{1,1}(10,:)'"/1 -> dotprod10/1
  dotprod10/1 -> Mux/10
  "IW{1,1}(11,:)'"/1 -> dotprod11/1
  dotprod11/1 -> Mux/11
  "IW{1,1}(12,:)'"/1 -> dotprod12/1
  dotprod12/1 -> Mux/12
  "IW{1,1}(13,:)'"/1 -> dotprod13/1
  dotprod13/1 -> Mux/13
  "IW{1,1}(14,:)'"/1 -> dotprod14/1
  dotprod14/1 -> Mux/14
  "IW{1,1}(15,:)'"/1 -> dotprod15/1
  dotprod15/1 -> Mux/15
  "IW{1,1}(16,:)'"/1 -> dotprod16/1
  dotprod16/1 -> Mux/16
  "IW{1,1}(17,:)'"/1 -> dotprod17/1
  dotprod17/1 -> Mux/17
  "IW{1,1}(18,:)'"/1 -> dotprod18/1
  dotprod18/1 -> Mux/18
  "IW{1,1}(19,:)'"/1 -> dotprod19/1
  dotprod19/1 -> Mux/19
  "IW{1,1}(20,:)'"/1 -> dotprod20/1
  dotprod20/1 -> Mux/20
  "IW{1,1}(21,:)'"/1 -> dotprod21/1
  dotprod21/1 -> Mux/21
  "IW{1,1}(22,:)'"/1 -> dotprod22/1
  dotprod22/1 -> Mux/22
  "IW{1,1}(23,:)'"/1 -> dotprod23/1
  dotprod23/1 -> Mux/23
  "IW{1,1}(24,:)'"/1 -> dotprod24/1
  dotprod24/1 -> Mux/24
  "IW{1,1}(25,:)'"/1 -> dotprod25/1
  dotprod25/1 -> Mux/25
  "IW{1,1}(26,:)'"/1 -> dotprod26/1
  dotprod26/1 -> Mux/26
  "IW{1,1}(27,:)'"/1 -> dotprod27/1
  dotprod27/1 -> Mux/27
  "IW{1,1}(28,:)'"/1 -> dotprod28/1
  dotprod28/1 -> Mux/28
  "IW{1,1}(29,:)'"/1 -> dotprod29/1
  dotprod29/1 -> Mux/29
  "IW{1,1}(30,:)'"/1 -> dotprod30/1
  dotprod30/1 -> Mux/30
  Mux/1 -> "iz{1,1}"/1

== system mrefrobotarm_modified_previous_y_previous_u_previous_ref_pert_2/m=0 sd=0.2/Layer 2/Delays 1 ==
  "p{2}" : Inport  PortDimensions=30
      mask Display: e = 0.06;c1 = [120 230 180]/255;c2 = ([120 230 180]+0)/(256+128);c3 = ([120 230 180]+128)/(256+128);patch([0 1 1 0],[0 0 1 1],c1);patch([0 1 1 1-e 1-e 0+e],[0 0 1 1-e 0+e 0+e],c2);patch([0 0 1 1-e 0+e 0+e],[0 1 1 1-e 1-e 0+e],c3);plot([0 1 1 0 0],[0 0 1 1 0]);
  mux : Mux  Inputs=1
      mask Display: e = 0.06;c1 = [120 150 230]/255;c2 = ([120 150 230]+0)/383;c3 = ([120 150 230]+128)/383;patch([0 1 1 0],[0 0 1 1],c1);patch([0 1 1 1-e 1-e 0+e],[0 0 1 1-e 0+e 0+e],c2);patch([0 0 1 1-e 0+e 0+e],[0 1 1 1-e 1-e 0+e],c3);plot([0 1 1 0 0],[0 0 1 1 0]);disp('Mux')
  "pd{2,1}" : Outport
      mask Display: e = 0.06;c1 = [120 230 180]/255;c2 = ([120 230 180]+0)/(256+128);c3 = ([120 230 180]+128)/(256+128);patch([0 1 1 0],[0 0 1 1],c1);patch([0 1 1 1-e 1-e 0+e],[0 0 1 1-e 0+e 0+e],c2);patch([0 0 1 1-e 0+e 0+e],[0 1 1 1-e 1-e 0+e],c3);plot([0 1 1 0 0],[0 0 1 1 0]);
  wires:
  "p{2}"/1 -> mux/1
  mux/1 -> "pd{2,1}"/1
